simulink model "twowheelsplttest"  (R2015a)
settings: Solver=ode3  StartTime=0.0  StopTime=10.0  RelTol=1e-3
values from neighbouring files (symbols this model uses):
  db = 0.000976    [ABAG.m]
  dg = 0.001953    [ABAG.m]
  eb = 0.75    [ABAG.m]
  eg = 0.5    [ABAG.m]
undefined symbols (not defined in the file or in its folder): alpha, endx, l, marge, speed
settings Model: Creator=s141010  LastModifiedBy=s141010
settings DataIOCC: LimitDataPoints=off

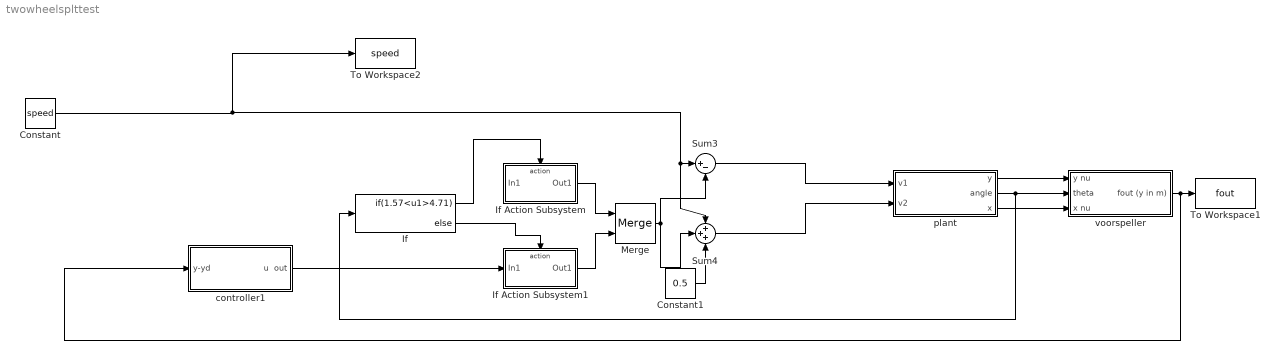
== system twowheelsplttest ==
  Constant : Constant  Value=speed
  Constant1 : Constant  Value=0.5
  If : If  IfExpression=1.57<u1>4.71
  If Action Subsystem : Subsystem  TreatAsAtomicUnit=on
  If Action Subsystem1 : Subsystem  TreatAsAtomicUnit=on
  Merge : Merge
  Sum3 : Sum  Inputs=|+-
  Sum4 : Sum  Inputs=3
  To Workspace1 : ToWorkspace  VariableName=fout  SaveFormat=Timeseries  SampleTime=-1
  To Workspace2 : ToWorkspace  VariableName=speed  SaveFormat=Timeseries  SampleTime=-1
  controller1 : Subsystem
  plant : Subsystem
  voorspeller : Subsystem
  wires:
  Sum3/1 -> plant/1(v1)
  voorspeller/1(fout (y in m)) -> controller1/1(y-yd), To Workspace1/1
  Constant/1 -> To Workspace2/1, Sum4/1, Sum3/1
  Sum4/1 -> plant/2(v2)
  If/2 -> If Action Subsystem1/Action
  If/1 -> If Action Subsystem/Action
  If Action Subsystem/1(Out1) -> Merge/1
  If Action Subsystem1/1(Out1) -> Merge/2
  plant/1(y) -> voorspeller/1(y nu)
  plant/3(x) -> voorspeller/3(x nu)
  plant/2(angle) -> voorspeller/2(theta), If/1
  controller1/1(u  out) -> If Action Subsystem1/1(In1)
  Merge/1 -> Sum4/2, Sum3/2
  Constant1/1 -> Sum4/3

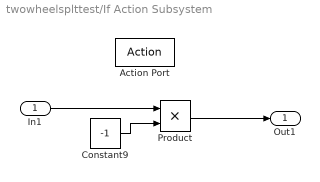
== system twowheelsplttest/If Action Subsystem ==
  In1 : Inport
  Action Port : ActionPort  ActionType=then
  Constant9 : Constant  Value=-1
  Product : Product
  Out1 : Outport
  wires:
  In1/1 -> Product/1
  Constant9/1 -> Product/2
  Product/1 -> Out1/1

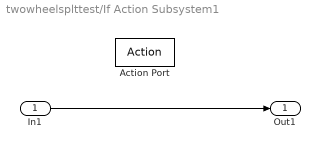
== system twowheelsplttest/If Action Subsystem1 ==
  In1 : Inport
  Action Port : ActionPort  ActionType=else
  Out1 : Outport
  wires:
  In1/1 -> Out1/1

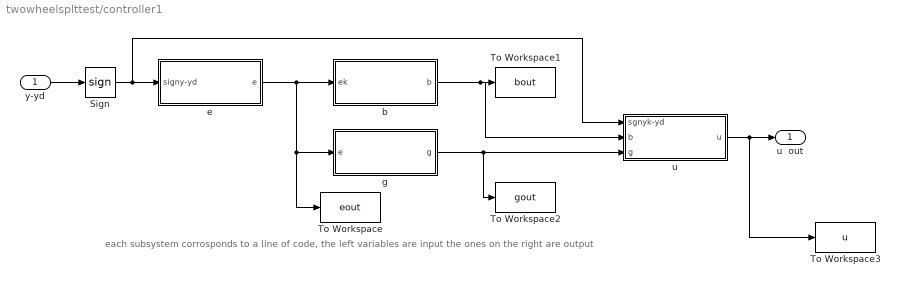
== system twowheelsplttest/controller1 ==
  note: each subsystem corrosponds to a line of code, the left variables are input the ones on the right are output
  y-yd : Inport
  Sign : Signum
  To Workspace : ToWorkspace  VariableName=eout  SaveFormat=Timeseries  SampleTime=-1
  To Workspace1 : ToWorkspace  VariableName=bout  SaveFormat=Timeseries  SampleTime=-1
  To Workspace2 : ToWorkspace  VariableName=gout  SaveFormat=Timeseries  SampleTime=-1
  To Workspace3 : ToWorkspace  VariableName=u  SaveFormat=Timeseries  SampleTime=-1
  b : Subsystem
  e : Subsystem
  g : Subsystem
  u : Subsystem
  u  out : Outport
  wires:
  y-yd/1 -> Sign/1
  Sign/1 -> u/1(sgnyk-yd), e/1(signy-yd)
  u/1(u) -> To Workspace3/1, u  out/1
  e/1(e) -> To Workspace/1, g/1(e), b/1(ek)
  b/1(b) -> u/2(b), To Workspace1/1
  g/1(g) -> To Workspace2/1, u/3(g)

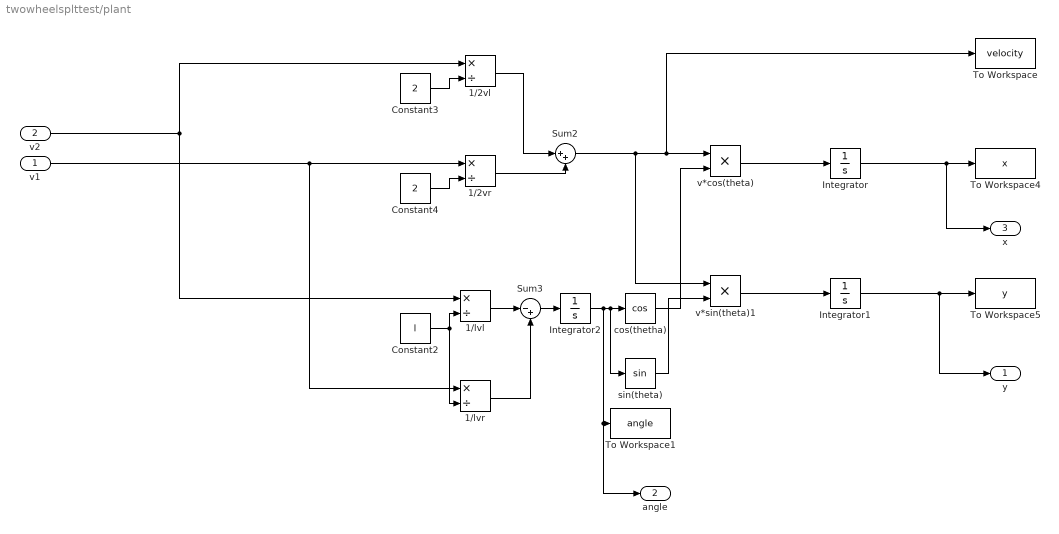
== system twowheelsplttest/plant ==
  v1 : Inport
  v2 : Inport  Port=2
  1/2vl : Product  Inputs=*/
  1/2vr : Product  Inputs=*/
  1/lvl : Product  Inputs=*/
  1/lvr : Product  Inputs=*/
  Constant2 : Constant  Value=l
  Constant3 : Constant  Value=2
  Constant4 : Constant  Value=2
  Integrator : Integrator
  Integrator1 : Integrator
  Integrator2 : Integrator
  Sum2 : Sum  Inputs=|++
  Sum3 : Sum  Inputs=|-+
  To Workspace : ToWorkspace  VariableName=velocity  SaveFormat=Timeseries  SampleTime=-1
  To Workspace1 : ToWorkspace  VariableName=angle  SaveFormat=Timeseries  SampleTime=-1
  To Workspace4 : ToWorkspace  VariableName=x  SampleTime=-1
  To Workspace5 : ToWorkspace  VariableName=y  SampleTime=-1
  cos(thetha) : Trigonometry  Operator=cos
  sin(theta) : Trigonometry
  v*cos(theta) : Product  Inputs=**
  v*sin(theta)1 : Product  Inputs=**
  y : Outport
  angle : Outport  Port=2
  x : Outport  Port=3
  wires:
  Constant3/1 -> 1/2vl/2
  Constant4/1 -> 1/2vr/2
  1/2vl/1 -> Sum2/1
  1/2vr/1 -> Sum2/2
  Constant2/1 -> 1/lvr/2, 1/lvl/2
  1/lvl/1 -> Sum3/1
  1/lvr/1 -> Sum3/2
  cos(thetha)/1 -> v*cos(theta)/2
  Sum2/1 -> v*sin(theta)1/1, To Workspace/1, v*cos(theta)/1
  v*cos(theta)/1 -> Integrator/1
  Integrator/1 -> x/1, To Workspace4/1
  sin(theta)/1 -> v*sin(theta)1/2
  v*sin(theta)1/1 -> Integrator1/1
  Integrator1/1 -> y/1, To Workspace5/1
  v2/1 -> 1/lvl/1, 1/2vl/1
  v1/1 -> 1/lvr/1, 1/2vr/1
  Sum3/1 -> Integrator2/1
  Integrator2/1 -> angle/1, To Workspace1/1, sin(theta)/1, cos(thetha)/1

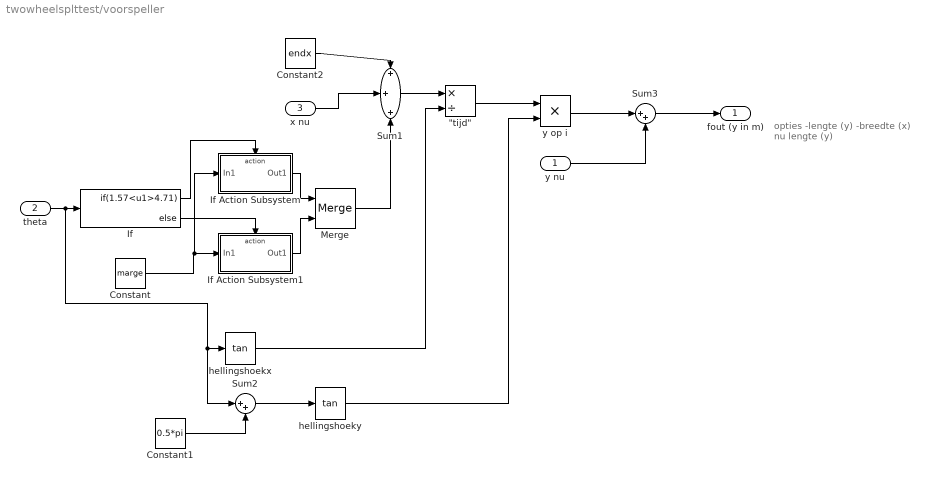
== system twowheelsplttest/voorspeller ==
  note: opties
      | -lengte  (y)
      | -breedte (x)
      |
      | nu
      | lengte (y)
  y nu : Inport
  theta : Inport  Port=2
  x nu : Inport  Port=3
  "\"tijd\"" : Product  Inputs=*/
  Constant : Constant  Value=marge
  Constant1 : Constant  Value=0.5*pi
  Constant2 : Constant  Value=endx
  If : If  IfExpression=1.57<u1>4.71
  If Action Subsystem : Subsystem  TreatAsAtomicUnit=on
  If Action Subsystem1 : Subsystem  TreatAsAtomicUnit=on
  Merge : Merge
  Sum1 : Sum  Inputs=3
  Sum2 : Sum  Inputs=|++
  Sum3 : Sum  Inputs=|++
  hellingshoekx : Trigonometry  Operator=tan  ApproximationMethod=CORDIC
  hellingshoeky : Trigonometry  Operator=tan  ApproximationMethod=CORDIC
  y op i : Product
  fout (y in m) : Outport
  wires:
  Merge/1 -> Sum1/3
  x nu/1 -> Sum1/2
  Constant2/1 -> Sum1/1
  Sum1/1 -> "\"tijd\""/1
  hellingshoekx/1 -> "\"tijd\""/2
  Constant1/1 -> Sum2/2
  Sum2/1 -> hellingshoeky/1
  hellingshoeky/1 -> y op i/2
  "\"tijd\""/1 -> y op i/1
  y op i/1 -> Sum3/1
  y nu/1 -> Sum3/2
  Sum3/1 -> fout (y in m)/1
  theta/1 -> If/1, Sum2/1, hellingshoekx/1
  If/1 -> If Action Subsystem/Action
  If/2 -> If Action Subsystem1/Action
  Constant/1 -> If Action Subsystem1/1(In1), If Action Subsystem/1(In1)
  If Action Subsystem/1(Out1) -> Merge/1
  If Action Subsystem1/1(Out1) -> Merge/2

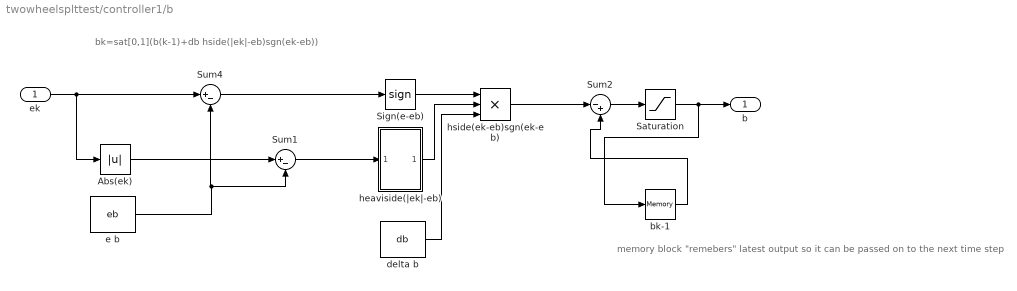
== system twowheelsplttest/controller1/b ==
  note: bk=sat[0,1](b(k-1)+db hside(|ek|-eb)sgn(ek-eb))
  note: memory block "remebers" latest output so it can be passed on to the next time step
  ek : Inport
  Abs(ek) : Abs
  Saturation : Saturate  UpperLimit=1  LowerLimit=-1
  Sign(e-eb) : Signum
  Sum1 : Sum  Inputs=|+-
  Sum2 : Sum  Inputs=|-+
  Sum4 : Sum  Inputs=|+-
  bk-1 : Memory
  delta b : Constant  Value=db
  e b : Constant  Value=eb
  heaviside(|ek|-eb) : Subsystem
  hside(ek-eb)sgn(ek-eb) : Product  Inputs=3
  b : Outport
  wires:
  ek/1 -> Abs(ek)/1, Sum4/1
  Sum4/1 -> Sign(e-eb)/1
  e b/1 -> Sum4/2, Sum1/2
  Sum1/1 -> heaviside(|ek|-eb)/1(In1)
  Abs(ek)/1 -> Sum1/1
  Sign(e-eb)/1 -> hside(ek-eb)sgn(ek-eb)/1
  heaviside(|ek|-eb)/1(Out1) -> hside(ek-eb)sgn(ek-eb)/2
  delta b/1 -> hside(ek-eb)sgn(ek-eb)/3
  hside(ek-eb)sgn(ek-eb)/1 -> Sum2/1
  Sum2/1 -> Saturation/1
  bk-1/1 -> Sum2/2
  Saturation/1 -> bk-1/1, b/1

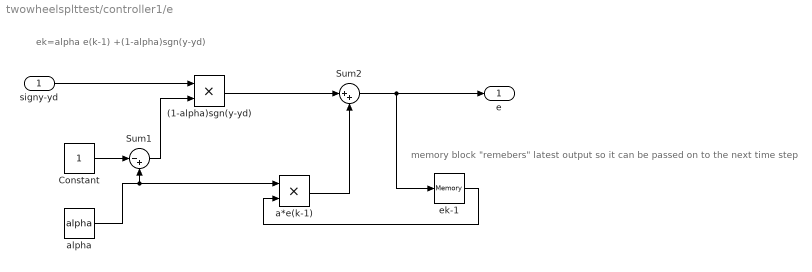
== system twowheelsplttest/controller1/e ==
  note: ek=alpha e(k-1) +(1-alpha)sgn(y-yd)
  note: memory block "remebers" latest output so it can be passed on to the next time step
  signy-yd : Inport
  (1-alpha)sgn(y-yd) : Product
  Constant : Constant
  Sum1 : Sum  Inputs=|-+
  Sum2 : Sum  Inputs=|++
  a*e(k-1) : Product
  alpha : Constant  Value=alpha
  ek-1 : Memory
  e : Outport
  wires:
  Sum1/1 -> (1-alpha)sgn(y-yd)/2
  Constant/1 -> Sum1/1
  alpha/1 -> a*e(k-1)/1, Sum1/2
  (1-alpha)sgn(y-yd)/1 -> Sum2/1
  signy-yd/1 -> (1-alpha)sgn(y-yd)/1
  a*e(k-1)/1 -> Sum2/2
  Sum2/1 -> ek-1/1, e/1
  ek-1/1 -> a*e(k-1)/2

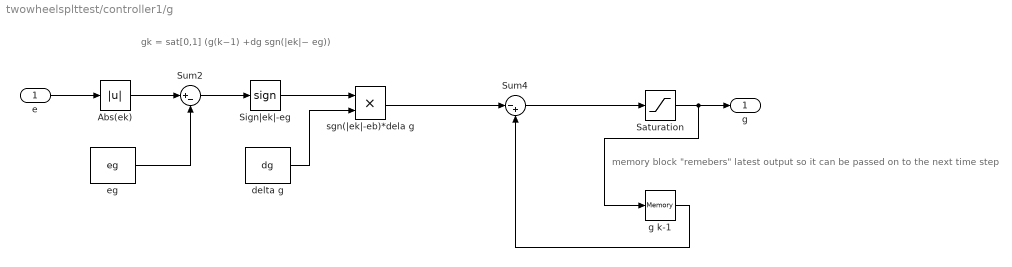
== system twowheelsplttest/controller1/g ==
  note: gk = sat[0,1] (g(k−1) +dg sgn(|ek|− eg))
  note: memory block "remebers" latest output so it can be passed on to the next time step
  e : Inport
  Abs(ek) : Abs
  Saturation : Saturate  UpperLimit=1  LowerLimit=-1
  Sign|ek|-eg : Signum
  Sum2 : Sum  Inputs=|+-
  Sum4 : Sum  Inputs=|-+
  delta g : Constant  Value=dg
  eg : Constant  Value=eg
  g k-1 : Memory
  sgn(|ek|-eb)*dela g : Product
  g : Outport
  wires:
  e/1 -> Abs(ek)/1
  Sum2/1 -> Sign|ek|-eg/1
  Saturation/1 -> g k-1/1, g/1
  Abs(ek)/1 -> Sum2/1
  eg/1 -> Sum2/2
  Sign|ek|-eg/1 -> sgn(|ek|-eb)*dela g/1
  delta g/1 -> sgn(|ek|-eb)*dela g/2
  sgn(|ek|-eb)*dela g/1 -> Sum4/1
  Sum4/1 -> Saturation/1
  g k-1/1 -> Sum4/2

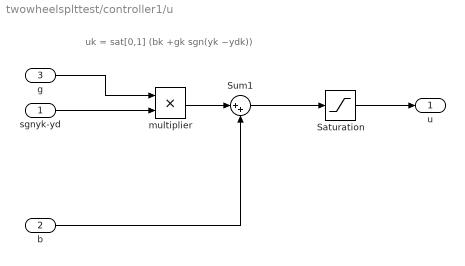
== system twowheelsplttest/controller1/u ==
  note: uk = sat[0,1] (bk +gk sgn(yk −ydk))
  sgnyk-yd : Inport
  b : Inport  Port=2
  g : Inport  Port=3
  Saturation : Saturate  UpperLimit=1  LowerLimit=-1
  Sum1 : Sum  Inputs=|++
  "multiplier " : Product
  u : Outport
  wires:
  sgnyk-yd/1 -> "multiplier "/2
  "multiplier "/1 -> Sum1/1
  g/1 -> "multiplier "/1
  Sum1/1 -> Saturation/1
  b/1 -> Sum1/2
  Saturation/1 -> u/1

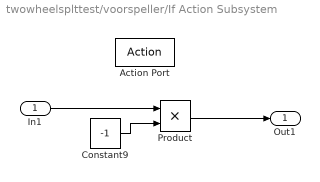
== system twowheelsplttest/voorspeller/If Action Subsystem ==
  In1 : Inport
  Action Port : ActionPort  ActionType=then
  Constant9 : Constant  Value=-1
  Product : Product
  Out1 : Outport
  wires:
  In1/1 -> Product/1
  Constant9/1 -> Product/2
  Product/1 -> Out1/1

== system twowheelsplttest/voorspeller/If Action Subsystem1 ==
  In1 : Inport
  Action Port : ActionPort  ActionType=else
  Out1 : Outport
  wires:
  In1/1 -> Out1/1

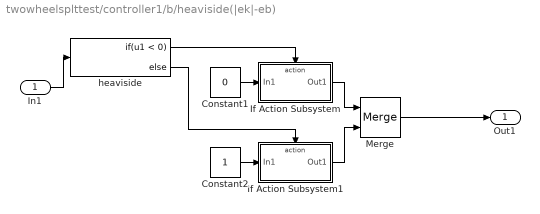
== system twowheelsplttest/controller1/b/heaviside(|ek|-eb) ==
  In1 : Inport
  Constant1 : Constant  Value=0
  Constant2 : Constant
  If Action Subsystem : Subsystem  TreatAsAtomicUnit=on
  If Action Subsystem1 : Subsystem  TreatAsAtomicUnit=on
  Merge : Merge
  heaviside : If  IfExpression=u1 < 0
  Out1 : Outport
  wires:
  If Action Subsystem1/1(Out1) -> Merge/2
  Constant1/1 -> If Action Subsystem/1(In1)
  Constant2/1 -> If Action Subsystem1/1(In1)
  Merge/1 -> Out1/1
  If Action Subsystem/1(Out1) -> Merge/1
  heaviside/1 -> If Action Subsystem/Action
  heaviside/2 -> If Action Subsystem1/Action
  In1/1 -> heaviside/1

== system twowheelsplttest/controller1/b/heaviside(|ek|-eb)/If Action Subsystem ==
  In1 : Inport
  Action Port : ActionPort  ActionType=then
  Out1 : Outport
  wires:
  In1/1 -> Out1/1

== system twowheelsplttest/controller1/b/heaviside(|ek|-eb)/If Action Subsystem1 ==
  In1 : Inport
  Action Port : ActionPort  ActionType=else
  Out1 : Outport
  wires:
  In1/1 -> Out1/1
